simulink model "inline_linearized"  (Simulink 7.4)
settings: Solver=ode45  StartTime=0.0  StopTime=100  FixedStep=0.05  RelTol=1e-3
InitFcn:
  | MpcSetup_linearized
values from neighbouring files (symbols this model uses):
  x_init_lin = [0.898 ... (first row only)    [MpcSetup.m]    (also in MpcSetup_linearized.m; compressor_setup.m; setup_compressor.m; test2.m = [0.899; 1.125; 0.1512; 440.7; 0])
settings Model: Creator=chkajon  LastModifiedBy=chkajon
settings SFSimCC: SimUserSources=../call_qpoases_m/call_qpoases.c
settings SFSimCC: SimUserIncludeDirs=|
  | ../call_qpoases_m/qpoases3/src
  | ../call_qpoases_m/qpoases3/include

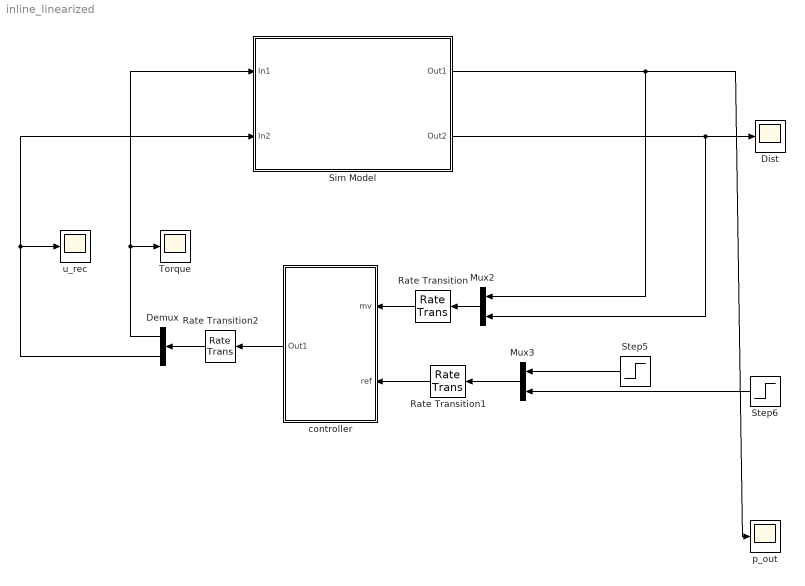
== system inline_linearized ==
  Demux : Demux  Outputs=2
  Dist : Scope
      settings: TimeRange=5  YMax=55  SaveName=SD  DataFormat=Array
  Mux2 : Mux  Inputs=2
  Mux3 : Mux  Inputs=2
  Rate Transition : RateTransition  X0=[1.126; 0.046]
  Rate Transition1 : RateTransition
  Rate Transition2 : RateTransition
  Sim Model : Subsystem
  Step5 : Step  Time=0  After=0  SampleTime=0
  Step6 : Step  Time=30  After=0  SampleTime=0
  Torque : Scope
      settings: TimeRange=30  YMin=-0.25  YMax=0.35  SaveName=ScopeData17
  controller : Subsystem
  p_out : Scope
      settings: TimeRange=20  YMin=0.17  YMax=0.187  SaveName=p_out  DataFormat=Array
  u_rec : Scope
      settings: TimeRange=5  YMin=-0.1  YMax=1.1
  wires:
  Step5/1 -> Mux3/1
  Step6/1 -> Mux3/2
  Demux/1 -> Torque/1, Sim Model/1(In1)
  controller/1(Out1) -> Rate Transition2/1
  Mux2/1 -> Rate Transition/1
  Mux3/1 -> Rate Transition1/1
  Rate Transition/1 -> controller/1(mv)
  Rate Transition1/1 -> controller/2(ref)
  Rate Transition2/1 -> Demux/1
  Demux/2 -> Sim Model/2(In2), u_rec/1
  Sim Model/2(Out2) -> Mux2/2, Dist/1
  Sim Model/1(Out1) -> p_out/1, Mux2/1

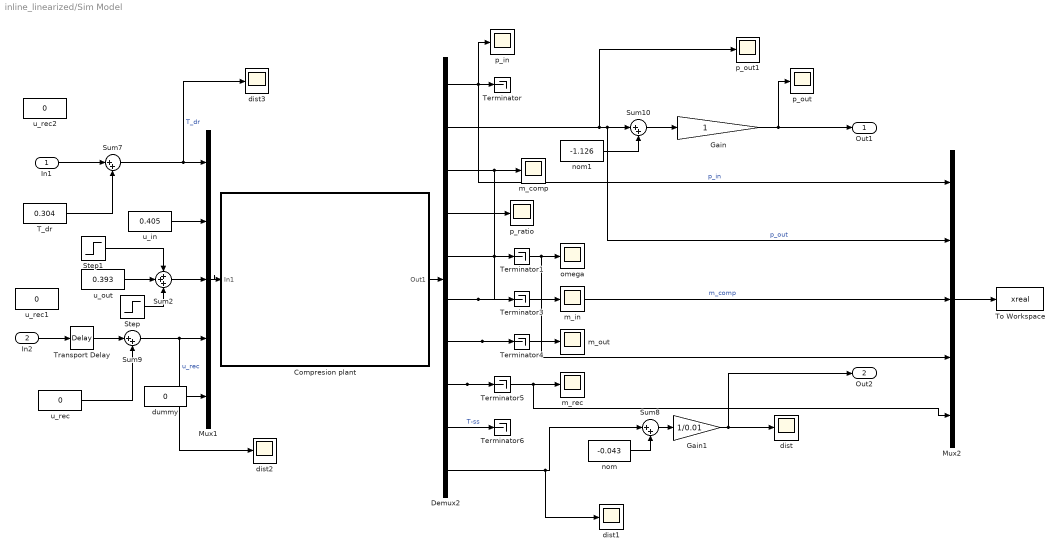
== system inline_linearized/Sim Model ==
  In1 : Inport
  In2 : Inport  Port=2
  Compresion plant : Subsystem
      mask Display: image(imread('comp_plant.jpg'))
  Demux2 : Demux  Outputs=10
  Gain : Gain
  Gain1 : Gain  Gain=1/0.01
  Mux1 : Mux  Inputs=5
  Mux2 : Mux  Inputs=5
  Step : Step  Time=10  After=0  SampleTime=0
  Step1 : Step  Time=100  After=0  SampleTime=0
  Sum{7..10} (4 alike) : Sum  Inputs=|++
  Sum2 : Sum  Inputs=+++
  T_dr : Constant  Value=0.304
  Terminator{,1,3..6} (6 alike) : Terminator
  To Workspace : ToWorkspace  VariableName=xreal  SampleTime=-1  SaveFormat=Structure With Time
  Transport Delay : TransportDelay
  dist{,1..3} (4 alike) : Scope
      dist settings: YMin=0.16552  YMax=0.1657  SaveName=ScopeData6
      dist1 settings: TimeRange=100  YMin=0.03  YMax=0.075  SaveName=ScopeData5
      dist2 settings: TimeRange=5  YMin=-0.25  YMax=1  SaveName=ScopeData4
      dist3 settings: TimeRange=100  YMin=-9  YMax=1  SaveName=ScopeData2
  dummy : Constant  Value=0
  m_comp : Scope
      settings: TimeRange=100  YMin=0.5  YMax=0.825  SaveName=m_comp  DataFormat=Array
  m_in : Scope
      settings: TimeRange=100  YMin=100.8  YMax=100.975  SaveName=ScopeData11
  m_out : Scope
      settings: TimeRange=100  YMin=100.8  YMax=100.975  SaveName=ScopeData12
  m_rec : Scope
      settings: TimeRange=100  YMin=100.8  YMax=100.975  SaveName=ScopeData13
  nom : Constant  Value=-0.043
  nom1 : Constant  Value=-1.126
  omega : Scope
      settings: TimeRange=100  YMin=200  YMax=700  SaveName=ScopeData10
  p_in : Scope
      settings: TimeRange=20  YMin=0.85  YMax=0.905  SaveName=ScopeData9
  p_out : Scope
      settings: TimeRange=100  YMin=-2.5  YMax=40  SaveName=ScopeData7
  p_out1 : Scope
      settings: TimeRange=100  YMin=100.8  YMax=100.975  SaveName=ScopeData8
  p_ratio : Scope
      settings: TimeRange=100  YMin=0.5  YMax=0.825  SaveName=p_ratio  DataFormat=Array
  u_in : Constant  Value=0.405
  u_out : Constant  Value=0.393
  u_rec : Constant  Value=0
  u_rec1 : Constant  Value=0
  u_rec2 : Constant  Value=0
  Out1 : Outport
  Out2 : Outport  Port=2
  wires:
  Demux2/9 -> Terminator6/1  "T-ss"
  Sum2/1 -> Mux1/3
  Step/1 -> Sum2/3
  Transport Delay/1 -> Sum9/1
  dummy/1 -> Mux1/5
  Demux2/10 -> dist1/1, Sum8/1
  Gain1/1 -> dist/1, Out2/1
  u_rec/1 -> Sum9/2
  T_dr/1 -> Sum7/2
  Gain/1 -> p_out/1, Out1/1
  nom1/1 -> Sum10/2
  Sum10/1 -> Gain/1
  Demux2/4 -> p_ratio/1
  Demux2/5 -> Terminator1/1, omega/1, Mux2/4
  Demux2/1 -> p_in/1, Terminator/1, Mux2/1  "p_in"
  Demux2/2 -> p_out1/1, Sum10/1, Mux2/2  "p_out"
  Sum8/1 -> Gain1/1
  nom/1 -> Sum8/2
  Sum9/1 -> dist2/1, Mux1/4  "u_rec"
  Sum7/1 -> Mux1/1, dist3/1  "T_dr"
  u_out/1 -> Sum2/2
  Demux2/7 -> m_out/1, Terminator4/1
  Demux2/8 -> Terminator5/1, m_rec/1, Mux2/5
  Demux2/6 -> m_in/1, Terminator3/1
  u_in/1 -> Mux1/2
  Demux2/3 -> m_comp/1, Mux2/3  "m_comp"
  Mux1/1 -> Compresion plant/1(In1)
  Compresion plant/1(Out1) -> Demux2/1
  Step1/1 -> Sum2/1
  Mux2/1 -> To Workspace/1
  In1/1 -> Sum7/1
  In2/1 -> Transport Delay/1

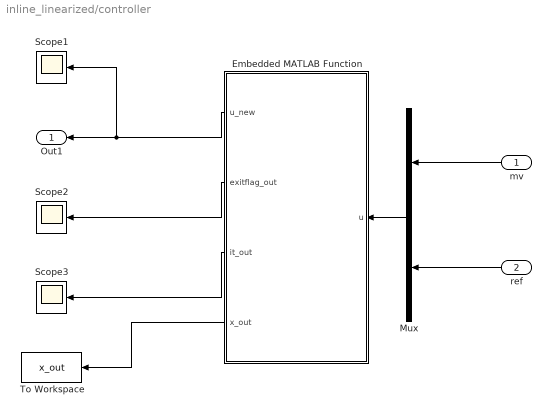
== system inline_linearized/controller ==
  mv : Inport
  ref : Inport  Port=2
  Embedded MATLAB Function : Stateflow chart  TreatAsAtomicUnit=on  SystemSampleTime=0.05
  Mux : Mux  Inputs=2
  Scope1 : Scope
      settings: YMin=0  YMax=0.6
  Scope2 : Scope
      settings: YMin=-1  YMax=1  SaveName=ScopeData15
  Scope3 : Scope
      settings: YMin=10  YMax=47.5  SaveName=ScopeData16
  To Workspace : ToWorkspace  VariableName=x_out  SampleTime=-1  SaveFormat=Structure With Time
  Out1 : Outport
  wires:
  mv/1 -> Mux/1
  Mux/1 -> Embedded MATLAB Function/1(u)
  ref/1 -> Mux/2
  Embedded MATLAB Function/1(u_new) -> Out1/1, Scope1/1
  Embedded MATLAB Function/3(it_out) -> Scope3/1
  Embedded MATLAB Function/2(exitflag_out) -> Scope2/1
  Embedded MATLAB Function/4(x_out) -> To Workspace/1

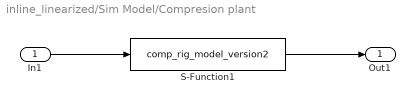
== system inline_linearized/Sim Model/Compresion plant ==
  In1 : Inport
  S-Function1 : S-Function  FunctionName=comp_rig_model_version2  Parameters=[], x_init_lin  EnableBusSupport=off
  Out1 : Outport
  wires:
  In1/1 -> S-Function1/1
  S-Function1/1 -> Out1/1

== matlab function controller/Embedded MATLAB Function ==
  data: u input double; u_new output double; exitflag_out output double; it_out output double; x_out output double
function [u_new,exitflag_out,it_out,x_out]  = fcn(u)
%#eml
% persistent C_new M LB UB Ga Gb Gc H Ain b A B upast xinit
persistent M LB UB Ain b upast xinit dxaug y_old C %x_init_lin
eml.extrinsic('disp');
eml.extrinsic('toc');
eml.extrinsic('tic');
eml.extrinsic('num2str');
eml.extrinsic('keyboard');
eml.extrinsic('quadprog');
% eml.extrinsic('call_qpoases_m');

p = 100;
m = 2;

if isempty(M)
    tic
    option = 1;
%     [H,C_new,M,UB,LB,b,Ain,Ga,Gb,Gc,xinit,upast] = get_matrices(option);
    [C,M,UB,LB,b,Ain,xinit,upast] = get_constant_matrices();
    dxaug = zeros(size(xinit));
    y_old = [0; 0];
    time = toc;
    disp(['Preparation time: ' num2str(time)]);
end

y = u(1:2);
% y(1) = y(1) + 1.126;
% y(2) = y(2) + 4.3;

% Estimate state info
dxaug = dxaug + M*(y - y_old - C*(dxaug));
xinit(1:5) = xinit(1:5) + dxaug(1:5);
xinit(6:end) = dxaug(6:end);
x_out = xinit;

yref = u(3:4) - dxaug(end-1:end);
% yref(1) = yref(1) + 1.126;
% yref(2) = yref(2) + 4.3;

% Get matrices - linearize about delayed rec.open input
% [A,B,C,H,Ga,Gb,Gc,df0,Sx,Su,Sf,UWT] = get_qp_matrices(xinit,[upast(1); dxaug(6)]);
[A,B,C,H,Ga,Gb,Gc,df0,Sx,Su,Sf,UWT] = get_qp_matrices(xinit,upast);

% df0=0*df0;


% Get reference and input vector
ysize = 2;
usize = 2;
Yref = zeros(p*ysize,1);
Upast = zeros(m*usize,1);
for i=1:p
    Yref(1+(i-1)*ysize:i*ysize,1) = yref - y;
end
for i=1:m
    % use delayed recycle opening as reference input
    Upast(1+(i-1)*usize,1) = upast(1);
    Upast(i*usize,1) = upast(2);
%     Upast(i*usize,1) = xinit(6);
end

% Update bounds
LBa = LB - Upast;
UBa = UB - Upast;

% Calculate initial state
% dx0 = [zeros(5,1); xinit(6:end-2)-xinit(6); xinit(end-1:end)];
dx0 = [zeros(5,1); xinit(6:end-2)-upast(2); xinit(end-1:end)];

% Gradient vector
f = df0'*Gc - Yref'*Ga + dx0'*Gb + Upast'*UWT;

% Solve QP
lbA = -inf(size(Ain,1),1);
[usol,cost,exitflag,it,lambda] = call_qpoases_m(H,f,Ain,LBa,UBa,lbA,b);
exitflag_out = exitflag(1,1);
it_out = it(1,1);

if exitflag_out~=0
    usol=quadprog(H,f,[eye(4); -eye(4); Ain],[UBa; -LBa; b]);
    exitflag_out
%     usol = zeros(4,1);
end

% tol = 1e-3;
% if (usol(1) < LBa(1)-tol || usol(2) < LBa(2)-tol || usol(1) > UBa(1)+tol || usol(2) > UBa(2)+tol)
%     usol
% end

% Apply next input
delta_u = usol(1:usize,1);
% u_new = [upast(1); dxaug(6)] + delta_u;
u_new = upast + delta_u;

% value of x about which we linearized
xlin = dxaug;
% xlin(6) = xinit(6);
xlin(6) = upast(2);
xlin(7:end) = 0;

dxaug = B*[u_new(1)-upast(1);u_new(2)] + A*(dxaug-xlin) + df0;

upast = u_new;


% % p=200;
% % m=8;
% p = 100;
% m = 2;
% 
% if isempty(M)
%     tic
%     option = 1;
% %     [H,C_new,M,UB,LB,b,Ain,Ga,Gb,Gc,xinit,upast] = get_matrices(option);
%     [C,M,UB,LB,b,Ain,xinit,upast,deltax] = get_constant_matrices();
% %     x_init_lin = [0.8980 1.1260 0.1500 439.5000 0]';
%     time = toc;
%     disp(['Preparation time: ' num2str(time)]);
% end
% 
% % tic
% 
% y=u(1:2);
% yref=u(3:4);
% 
% 
% %%%%%%%%%%%%%%%%%%%%%%%%%%%%%%%%%%%%%%%%%%%%%%%%%%%%%%%%%%
% 
% 
% % estimate the state information
% 
% 
% % xinit  = xinit + M*(y - C_new*xinit);
% deltax = deltax + M*(y - C*deltax);
% xinit = deltax + xinit;
% x_out = xinit;
% 
% [A,B,C,H,Ga,Gb,Gc] = get_qp_matrices(xinit,upast);
% 
% %%%%%%%%%%%%%%%%%%%%%%%%%%%%%%%%%%%%%%%%%%%%%%%%%%%%%%%%%%
% 
% 
% 
% % upper and lower bounds wrt past input
% Upast = zeros(m*2,1);
% 
% for i=1:m
%     Upast(1+(i-1)*2:i*2,1)=upast;
% end
% 
% LBa=LB-Upast;
% UBa=UB-Upast;
% 
% 
% 
% %%%%%%%%%%%%%%%%%%%%%%%%%%%%%%%%%%%%%%%%%%%%%%%%%%%%%%%%%%
% 
% % generate the output reference vector
% 
% R = zeros(p*2,1);
% 
% for i=1:p
% %     R(1+(i-1)*2:i*2,1)=yref - y;
%     R(1+(i-1)*2:i*2,1)=y - yref;
% end
% 
% % generate the gradient vector
% 
% % f = deltax'*Gb+Upast'*Gc-R'*Ga;
% f = deltax'*Gb-R'*Ga;
% 
% % xinit1 = xinit;
% % upast1 = upast;
% 
% lbA = -inf(size(Ain,1),1);
% ubA = b;
% [usol,cost,exitflag,it,lambda] = call_qpoases_m(H,f,Ain,LBa,UBa,lbA,ubA);
% exitflag_out = exitflag(1,1);
% it_out = it(1,1);
% dunext=usol(1:2,1);
% 
% deltax= A*deltax + B*(dunext);
% 
% u_new = dunext + upast;
% % u_new = zeros(2,1);
% 
% upast = u_new;

% time2 = toc;
% disp(['Normal Execution Time: ' num2str(time2)]);
%%%%%%%%%%%%%%%%%%%%%%%%%%%%%%%%%%%%%%%%%%%%%%%%%%%%%%%%%%


% solve the QP

% usol=quadprog(H_qp,f,Ain,b,[],[],LBa,UBa);
% 
% 
% %%%%%%%%%%%%%%%%%%%%%%%%%%%%%%%%%%%%%%%%%%%%%%%%%%%%%%%%%%
% 
% 
% % extract the control moves for next time step
% 
% 
% dunext=usol(1:2,1);
% 
% 
% %%%%%%%%%%%%%%%%%%%%%%%%%%%%%%%%%%%%%%%%%%%%%%%%%%%%%%%%%%
% 
% 
% % initial conditions are updated
% 
% 
% xinit= A*xinit + B*(dunext+upast);
% 
% 
% %%%%%%%%%%%%%%%%%%%%%%%%%%%%%%%%%%%%%%%%%%%%%%%%%%%%%%%%%%
% 
% % control moves are sent to the plant
% 
% upast=dunext+upast;
% 
% sys=upast;
